simulink model "Single_Phase_Motor_SimArch"  (R2022b)
settings: Solver=FixedStepDiscrete  StartTime=0.0  StopTime=SimTime  FixedStep=Ts_SIM  RelTol=1e-3
PreLoadFcn:
  | clear mex;
  | clear all;
  | addpath(genpath('exe'));
  | addpath(genpath('exported_models'));
  | addpath(genpath('settings'));
  | addpath(genpath('source'));
  | addpath(genpath('tools'));
  | 
  | try
  | FMIKit.initialize()
  | catch
  | display('FMI Kit Initialization Skipped');
  | end
PostLoadFcn:
  | SPM_SimArch_Config;
  | SPM_SimArch_GUI;
undefined symbols (not defined in the file): freq, Ts_MCI_ZC, Ts_Model, Vmains
libraries: mciapi_libbrowser x1, pdb_libbrowser x1
CloseFcn:
  | rmpath(genpath('exe'));
  | rmpath(genpath('exported_models'));
  | rmpath(genpath('settings'));
  | rmpath(genpath('source'));
  | rmpath(genpath('tools'));
Description:
  | Main Model for Single Phase Motor Simulation Architecture
settings Model: Creator=BEDNASA  LastModifiedBy=HENRIE2
settings SolverCC: AlgebraicLoopSolver=TrustRegion
settings DebuggingCC: UnconnectedInputMsg=warning  UnconnectedOutputMsg=warning  UnconnectedLineMsg=warning  SFMachineParentedDataDiag=warning
settings ModelReferenceCC: EnableRefExpFcnMdlSchedulingChecks=on
settings RTWCC: CustomInclude="\"C:\\Data\\MBD_SPM_SimArch\\tools\\FMIKit\\FMIKit-Simulink-2.9\\include\""  CustomSource="\"C:\\Data\\MBD_SPM_SimArch\\tools\\FMIKit\\FMIKit-Simulink-2.9\\src\\FMU.cpp\" \"C:\\Data\\MBD_SPM_SimArch\\tools\\FMIKit\\FMIKit-Simulink-2.9\\src\\FMU1.cpp\" \"C:\\Data\\MBD_SPM_SimArch\\tools\\FMIKit\\FMIKit-Simulink-2.9\\src\\FMU2.cpp\""  DLArmComputeVersion=19.05

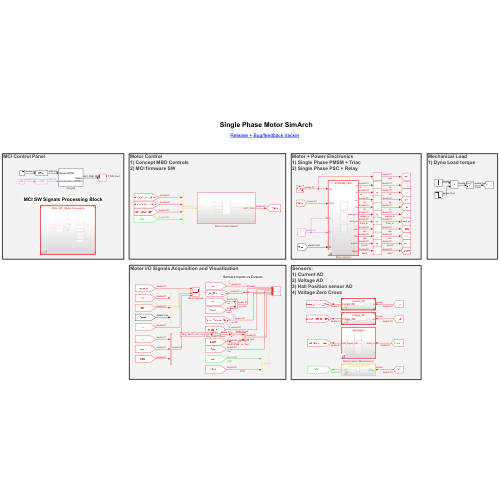
[thumbnail: Simulink's stored preview of the top-level diagram]
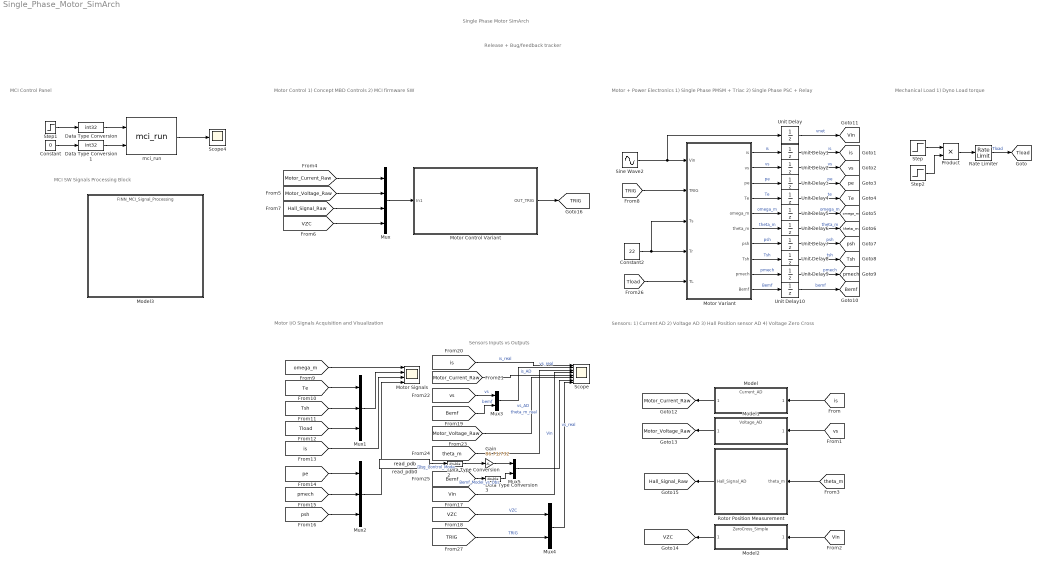
== system Single_Phase_Motor_SimArch ==
  note: Sensors Inputs vs Outputs
  note: MCI SW Signals Processing Block
  note: MCI Control Panel
  note: Release + Bug/feedback tracker
  note: Single Phase Motor SimArch
  note: Motor Control
      | 1) Concept MBD Controls
      | 2) MCI firmware SW
  note: Motor + Power Electronics
      | 1) Single Phase PMSM + Triac
      | 2) Single Phase PSC + Relay
  note: Mechanical Load
      | 1) Dyno Load torque
  note: Sensors:
      | 1) Current AD
      | 2) Voltage AD
      | 3) Hall Position sensor AD
      | 4) Voltage Zero Cross
  note: Motor I/O Signals Acquisition and Visualization
  Constant : Constant  Value=0
  Constant2 : Constant  Value=22
  Data Type Conversion : DataTypeConversion  OutDataTypeStr=int32  SaturateOnIntegerOverflow=off  RndMeth=Floor
  Data Type Conversion1 : DataTypeConversion  OutDataTypeStr=int32  SaturateOnIntegerOverflow=off  RndMeth=Floor
  Data Type Conversion2 : DataTypeConversion  OutDataTypeStr=double  SaturateOnIntegerOverflow=off  RndMeth=Floor
  Data Type Conversion3 : DataTypeConversion  OutDataTypeStr=double  SaturateOnIntegerOverflow=off  RndMeth=Floor
  Gain : Gain  Gain=86.71/732
  Model : ModelReference  ModelNameDialog=Current_AD.slx  SimulationMode=Normal  ModelReferenceVersion=6.0
  Model1 : ModelReference  ModelNameDialog=Voltage_AD.slx  SimulationMode=Normal  ModelReferenceVersion=6.0
  Model2 : ModelReference  ModelNameDialog=ZeroCross_Simple.slx  SimulationMode=Normal  ModelReferenceVersion=1.17
  Model3 : ModelReference  ModelNameDialog=FINN_MCI_Signal_Processing.slx  SimulationMode=Normal  ModelReferenceVersion=2.11
  Motor Control Variant : Subsystem
  Motor Signals : Scope  NumInputPorts=4
  Motor Variant : Subsystem  Variant=on  VariantActivationTime=code compile  PropagateVariantConditions=on
  Mux : Mux
  Mux1 : Mux  Inputs=3
  Mux2 : Mux  Inputs=3
  Mux3 : Mux  Inputs=2
  Mux4 : Mux  Inputs=2
  Mux5 : Mux  Inputs=2
  Product : Product
  Rate Limiter : RateLimiter  RisingSlewLimit=0.19  FallingSlewLimit=-0.01  SampleTimeMode=inherited
  Rotor Position Measurement : Subsystem  Variant=on  VariantActivationTime=code compile  PropagateVariantConditions=on
  Scope : Scope  NumInputPorts=8
  Scope4 : Scope
  Sine Wave2 : Sin  Amplitude=Vmains*sqrt(2)  Frequency=2*pi*freq  SampleTime=Ts_Model
  Step : Step  Time=0.60  Before=-0.01*0  After=0.081*0.6  SampleTime=0
  Step1 : Step  Time=0.5  After=500  SampleTime=0
  Step2 : Step  Time=60  Before=1  After=0  SampleTime=0
  Unit Delay{,1..10} (11 alike) : UnitDelay  SampleTime=-1  HasFrameUpgradeWarning=on
  mci_run : mciapi_libbrowser/mci_run  SFunctionModules=''
      settings: SourceProductName=Sim Arch
  read_pdb0 : pdb_libbrowser/read_pdb  vstring=Dbg_bemf_volt_tmp
      settings: SourceProductName=Sim Arch
  tag scope: Bemf=global, Hall_Signal_Raw=global, Motor_Current_Raw=global, Motor_Voltage_Raw=global, TRIG=global, Te=global, Tload=global, Tsh=global, VZC=global, Vin=global, is=global, omega_m=global, pe=global, pmech=global, psh=global, theta_m=global, vs=global
  wires:
  Motor Variant/3(pe) -> Unit Delay3/1  "pe"
  Motor Variant/4(Te) -> Unit Delay4/1  "Te"
  Motor Variant/7(psh) -> Unit Delay7/1  "psh"
  Motor Variant/8(Tsh) -> Unit Delay8/1  "Tsh"
  Motor Variant/9(pmech) -> Unit Delay9/1  "pmech"
  Motor Variant/10(Bemf) -> Unit Delay10/1  "Bemf"
  [Motor_Current_Raw] -> Mux/1
  [Motor_Voltage_Raw] -> Mux/2
  Mux/1 -> Motor Control Variant/1(In1)
  Motor Control Variant/1(OUT_TRIG) -> [TRIG]
  [Tsh] -> Mux1/2
  [Tload] -> Mux1/3
  [Te] -> Mux1/1
  [pmech] -> Mux2/2
  [psh] -> Mux2/3
  [pe] -> Mux2/1
  [omega_m] -> Motor Signals/1
  Mux1/1 -> Motor Signals/2
  [is] -> Motor Signals/3
  Mux2/1 -> Motor Signals/4
  [is] -> Scope/1  "is_real"
  [Motor_Current_Raw] -> Scope/5  "is_AD"
  [theta_m] -> Scope/3  "theta_m_real"
  Rate Limiter/1 -> [Tload]  "Tload"
  [Hall_Signal_Raw] -> Mux/3
  [VZC] -> Mux/4
  Model/1 -> [Motor_Current_Raw]
  Model1/1 -> [Motor_Voltage_Raw]
  Rotor Position Measurement/1(Hall_Signal_AD) -> [Hall_Signal_Raw]
  [theta_m] -> Rotor Position Measurement/1(theta_m)
  [vs] -> Model1/1
  [is] -> Model/1
  Model2/1 -> [VZC]
  [Vin] -> Model2/1
  [Vin] -> Scope/4  "Vin"
  [vs] -> Mux3/1  "vs"
  [Bemf] -> Mux3/2  "bemf"
  [Motor_Voltage_Raw] -> Scope/6  "vs_AD"
  Mux3/1 -> Scope/2  "vs_real"
  Sine Wave2/1 -> Motor Variant/1(Vin), Unit Delay/1
  Constant2/1 -> Motor Variant/4(Tr), Motor Variant/3(Ts)
  [Tload] -> Motor Variant/5(TL)
  Step1/1 -> Data Type Conversion/1
  Constant/1 -> Data Type Conversion1/1
  mci_run/1 -> Scope4/1
  Data Type Conversion/1 -> mci_run/1
  Data Type Conversion1/1 -> mci_run/2
  [TRIG] -> Mux4/2  "TRIG"
  [VZC] -> Mux4/1  "VZC"
  Mux4/1 -> Scope/8
  [TRIG] -> Motor Variant/2(TRIG)
  Motor Variant/2(vs) -> Unit Delay2/1  "vs"
  Motor Variant/1(is) -> Unit Delay1/1  "is"
  Motor Variant/5(omega_m) -> Unit Delay5/1  "omega_m"
  Motor Variant/6(theta_m) -> Unit Delay6/1  "theta_m"
  Unit Delay/1 -> [Vin]  "vnet"
  Unit Delay1/1 -> [is]  "is"
  Unit Delay2/1 -> [vs]  "vs"
  Unit Delay3/1 -> [pe]  "pe"
  Unit Delay4/1 -> [Te]  "te"
  Unit Delay5/1 -> [omega_m]  "omega_m"
  Unit Delay6/1 -> [theta_m]  "theta_m"
  Unit Delay7/1 -> [psh]  "psh"
  Unit Delay8/1 -> [Tsh]  "tsh"
  Unit Delay9/1 -> [pmech]  "pmech"
  Unit Delay10/1 -> [Bemf]  "bemf"
  Step/1 -> Product/1
  Step2/1 -> Product/2
  Product/1 -> Rate Limiter/1
  Mux5/1 -> Scope/7  "vs_real"
  read_pdb0/1 -> Data Type Conversion2/1  "Dbg_Control_Mode"
  [Bemf] -> Data Type Conversion3/1  "Bemf_Model_vs_Obs"
  Data Type Conversion3/1 -> Mux5/2
  Gain/1 -> Mux5/1
  Data Type Conversion2/1 -> Gain/1

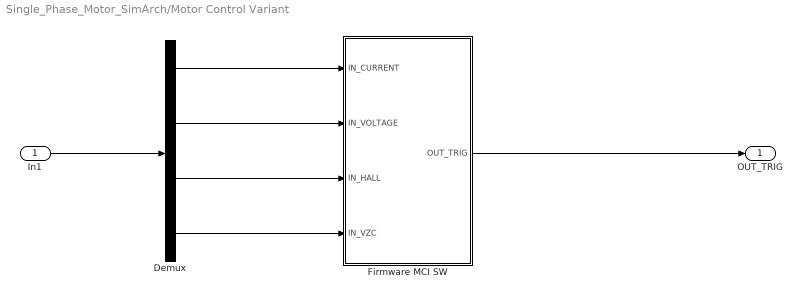
== system Single_Phase_Motor_SimArch/Motor Control Variant ==
  In1 : Inport
  Demux : Demux
  Firmware MCI SW : Subsystem
  OUT_TRIG : Outport
  wires:
  In1/1 -> Demux/1
  Demux/1 -> Firmware MCI SW/1(IN_CURRENT)
  Demux/2 -> Firmware MCI SW/2(IN_VOLTAGE)
  Demux/3 -> Firmware MCI SW/3(IN_HALL)
  Demux/4 -> Firmware MCI SW/4(IN_VZC)
  Firmware MCI SW/1(OUT_TRIG) -> OUT_TRIG/1

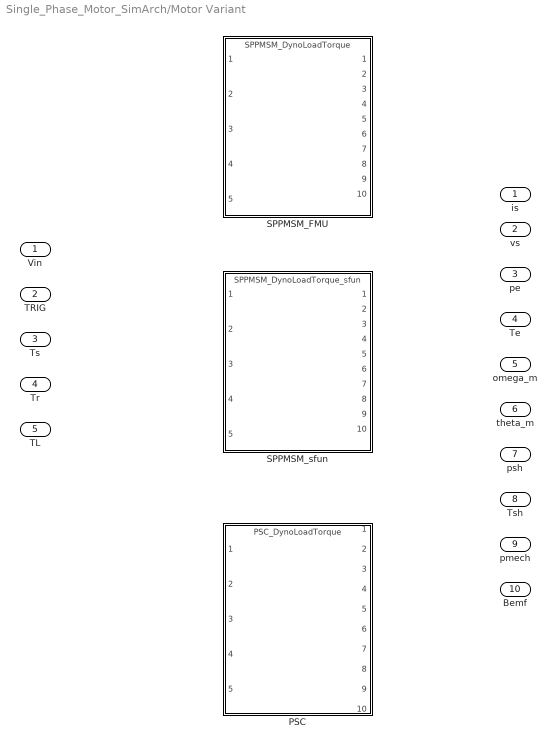
== system Single_Phase_Motor_SimArch/Motor Variant ==
  Vin : Inport
  TRIG : Inport  Port=2
  Ts : Inport  Port=3
  Tr : Inport  Port=4
  TL : Inport  Port=5
  PSC : ModelReference  ModelNameDialog=PSC_DynoLoadTorque.slx  SimulationMode=Normal  VariantControl=MotorType == 2  ModelReferenceVersion=6.1
  SPPMSM_FMU : ModelReference  DisableCoverage=on  ModelNameDialog=SPPMSM_DynoLoadTorque.slx  SimulationMode=Normal  VariantControl=MotorType == 11  ModelReferenceVersion=6.3
  SPPMSM_sfun : ModelReference  DisableCoverage=on  ModelNameDialog=SPPMSM_DynoLoadTorque_sfun.slx  SimulationMode=Normal  VariantControl=MotorType == 12  ModelReferenceVersion=6.1
  is : Outport
  vs : Outport  Port=2
  pe : Outport  Port=3
  Te : Outport  Port=4
  omega_m : Outport  Port=5
  theta_m : Outport  Port=6
  psh : Outport  Port=7
  Tsh : Outport  Port=8
  pmech : Outport  Port=9
  Bemf : Outport  Port=10

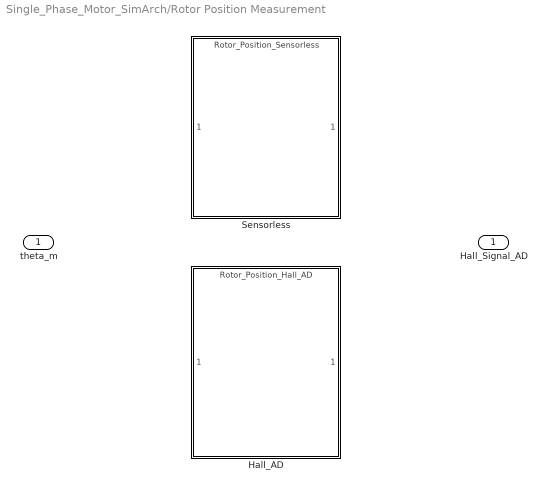
== system Single_Phase_Motor_SimArch/Rotor Position Measurement ==
  theta_m : Inport
  Hall_AD : ModelReference  ModelNameDialog=Rotor_Position_Hall_AD.slx  SimulationMode=Normal  VariantControl=Position_Sensor == 2  ModelReferenceVersion=1.21
  Sensorless : ModelReference  DisableCoverage=on  ModelNameDialog=Rotor_Position_Sensorless.slx  SimulationMode=Normal  VariantControl=Position_Sensor == 1  ModelReferenceVersion=1.20
  Hall_Signal_AD : Outport

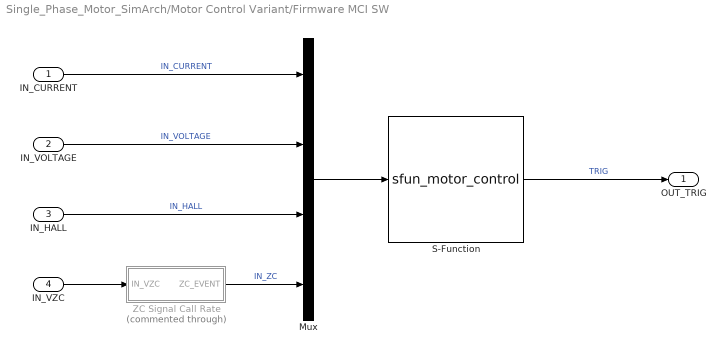
== system Single_Phase_Motor_SimArch/Motor Control Variant/Firmware MCI SW ==
  IN_CURRENT : Inport
  IN_VOLTAGE : Inport  Port=2
  IN_HALL : Inport  Port=3
  IN_VZC : Inport  Port=4
  Mux : Mux
  S-Function : S-Function  FunctionName=sfun_motor_control  Parameters=Ts_MCI_F  SFunctionDeploymentMode=off  EnableBusSupport=off
  ZC Signal Call Rate : Subsystem  Commented=through  TreatAsAtomicUnit=on  SystemSampleTime=Ts_MCI_ZC
  OUT_TRIG : Outport
  wires:
  Mux/1 -> S-Function/1
  IN_VZC/1 -> ZC Signal Call Rate/1(IN_VZC)
  IN_HALL/1 -> Mux/3  "IN_HALL"
  IN_VOLTAGE/1 -> Mux/2  "IN_VOLTAGE"
  IN_CURRENT/1 -> Mux/1  "IN_CURRENT"
  ZC Signal Call Rate/1(ZC_EVENT) -> Mux/4  "IN_ZC"
  S-Function/1 -> OUT_TRIG/1  "TRIG"

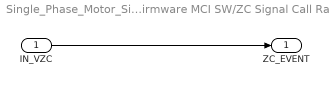
== system Single_Phase_Motor_SimArch/Motor Control Variant/Firmware MCI SW/ZC Signal Call Rate ==
  IN_VZC : Inport
  ZC_EVENT : Outport
  wires:
  IN_VZC/1 -> ZC_EVENT/1
